simulink library "LnrIntrpnDyn"  (R2013b)
settings: Solver=ode45  StartTime=0.0  StopTime=10.0  RelTol=1e-3
settings Model: Creator=qzwc4r  LastModifiedBy=qzwc4r

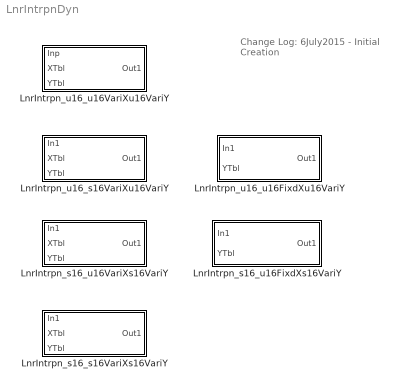
== system LnrIntrpnDyn ==
  note: Change Log:
      |
      | 6July2015
      | - Initial Creation
  LnrIntrpn_s16_s16VariXs16VariY : Subsystem  mask(LnrIntrpn_s16_s16VariXs16VariY){}
      mask help:
      | Linear interpolation with signed input and signed output (variable X axis)
      | XTbl and YTbl sizes must be equal.
      settings: AttributesFormatString=Lnr ( s16VariX , s16VariY )
      mask Display:
      | Xx = [0.3, .9];
      | Xy = [0.5, 0.5];
      | Yx = [0.6, 0.6];
      | Yy = [0.1, .9];
      | 
      | px = [.3, .4, .6, .7, .8, .9];
      | py = [.1,  .1, .25, .4, .5, .9];
      | plot(Xx,Xy, Yx,Yy, px,py)
      | 
      | port_label('input',1,'Inp')
      | port_label('input',2,'XTbl')
      | port_label('input',3,'YTbl')
  LnrIntrpn_s16_u16FixdXs16VariY : Subsystem  mask(LnrIntrpn_s16_u16FixdXs16VariY){DeltaX=[]}
      mask help: Linear interpolation with unsigned input and signed output (fixed X axis)
      settings: AttributesFormatString=Lnr ( u16FixdX , s16VariY )
      mask Display:
      | Xx = [0.3, .9];
      | Xy = [0.4, 0.4];
      | Yx = [0.3, 0.3];
      | Yy = [0, .9];
      | 
      | px = [0.3, .4, .5, .6, .8, .9];
      | py = [.75, .75, .6, .3, .1, .1];
      | 
      | %tic marks
      | tx1 = [0.3, 0.3];
      | tx2 = tx1 + 0.15;
      | tx3 = tx2 + 0.15;
      | tx4 = tx3 + 0.15;
      | tx5 = tx4 + 0.15;
      | ty = [.27, .53];
      | 
      | plot(Xx,Xy, Yx,Yy, px,py, tx1,ty, tx2,ty, tx3,ty, tx4,ty, tx5,ty)
      | 
      | port_label('input',1,'Inp')
      | port_label('input',2,'YTbl')
  LnrIntrpn_s16_u16VariXs16VariY : Subsystem  mask(LnrIntrpn_s16_u16VariXs16VariY){}
      mask help:
      | Linear interpolation with unsigned input and signed output (variable X axis)
      | XTbl and YTbl sizes must be equal.
      settings: AttributesFormatString=Lnr ( u16VariX , s16VariY )
      mask Display:
      | Xx = [0.3, .9];
      | Xy = [0.4, 0.4];
      | Yx = [0.3, 0.3];
      | Yy = [0, .9];
      | 
      | px = [0.3, .35, .4, .6, .8, .9];
      | py = [.75, .75, .7, .3, .1, .1];
      | plot(Xx,Xy, Yx,Yy, px,py)
      | 
      | port_label('input',1,'Inp')
      | port_label('input',2,'XTbl')
      | port_label('input',3,'YTbl')
  LnrIntrpn_u16_s16VariXu16VariY : Subsystem  mask(LnrIntrpn_u16_s16VariXu16VariY){}
      mask help:
      | Linear interpolation with signed input and unsigned output (variable X axis)
      | XTbl and YTbl sizes must be equal.
      settings: AttributesFormatString=Lnr ( s16VariX , u16VariY )
      mask Display:
      | Xx = [0.3, .9];
      | Xy = [.05, .05];
      | Yx = [.6, .6];
      | Yy = [.05, .9];
      | 
      | px = [0.3, .4, .5, .6, .7, .9];
      | py = [.15, .15, .25, .5, .6, .65];
      | plot(Xx,Xy, Yx,Yy, px,py)
      | 
      | port_label('input',1,'Inp')
      | port_label('input',2,'XTbl')
      | port_label('input',3,'YTbl')
  LnrIntrpn_u16_u16FixdXu16VariY : Subsystem  mask(LnrIntrpn_u16_u16FixdXu16VariY){DeltaX=[]}
      mask help: Linear interpolation with unsigned input and unsigned output (fixed X axis)
      settings: AttributesFormatString=Lnr ( u16FixdX , u16VariY )
      mask Display:
      | Xx = [0.3, .9];
      | Xy = [0.1, 0.1];
      | Yx = [0.3, 0.3];
      | Yy = [0.1, .9];
      | 
      | px = [0.3, .35, .4, .45, .5, .6, .8];
      | py = [0.1,  0.4, .6, .7, .75, .78, .8];
      | 
      | %tic marks
      | tx1 = [0.3, 0.3];
      | tx2 = tx1 + 0.15;
      | tx3 = tx2 + 0.15;
      | tx4 = tx3 + 0.15;
      | tx5 = tx4 + 0.15;
      | ty = [.1, .25];
      | 
      | plot(Xx,Xy, Yx,Yy, px,py, tx1,ty, tx2,ty, tx3,ty, tx4,ty, tx5,ty)
      | 
      | port_label('input',1,'Inp')
      | port_label('input',2,'YTbl')
  LnrIntrpn_u16_u16VariXu16VariY : Subsystem  mask(LnrIntrpn_u16_u16VariXu16VariY){}
      mask help:
      | Linear interpolation with unsigned input and unsigned output (variable X axis)
      | XTbl and YTbl sizes must be equal.
      settings: AttributesFormatString=Lnr ( u16VariX , u16VariY )
      mask Display:
      | Xx = [0.25, .9];
      | Xy = [0.1, 0.1];
      | Yx = [0.25, 0.25];
      | Yy = [0.1, .9];
      | 
      | px = [0.25, .3, .35, .4, .5, .6, .8];
      | py = [0.1,  0.4, .6, .7, .75, .78, .8];
      | plot(Xx,Xy, Yx,Yy, px,py)
      | 
      | port_label('input',1,'Inp')
      | port_label('input',2,'XTbl')
      | port_label('input',3,'YTbl')

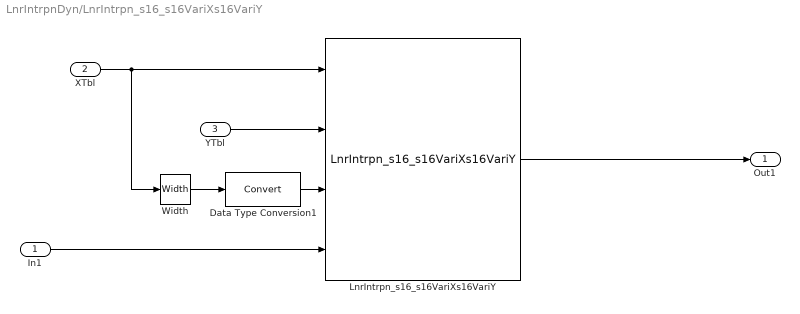
== system LnrIntrpnDyn/LnrIntrpn_s16_s16VariXs16VariY ==
  In1 : Inport
  XTbl : Inport  Port=2
  YTbl : Inport  Port=3
  Data Type Conversion1 : DataTypeConversion
  LnrIntrpn_s16_s16VariXs16VariY : S-Function  FunctionName=LnrIntrpn_s16_s16VariXs16VariY  EnableBusSupport=off  mask(Legacy Function){SFunctionSpec=int16 y1 = LnrIntrpn_s16_s16VariXs16VariY( int16 u1[],  int16 u2[], uint16 u3,  int16 u4), ShowSpec=on}
      mask prompts: ShowSpec "Display function specification"
      mask help:
      | This block allows you to call the legacy functions specified by the following Legacy Code Tool definition:
      | def.SFunctionName = 'LnrIntrpn_s16_s16VariXs16VariY';
      | def.OutputFcnSpec = ' int16 y1 = LnrIntrpn_s16_s16VariXs16VariY( int16 u1[],  int16 u2[], uint16 u3,  int16 u4)';
      | def.HeaderFiles = {'NxtrIntrpn.h', 'NxtrIntrpn_MemMap.h', 'Std_Types.h', 'Platform_Types.h', 'Compiler.h', 'Compiler_Cfg.h'};
      | def.SourceFiles = {'NxtrIntrpn.c'};
      | def.IncPaths = {'..\SrcFiles'};
      | def.SrcPaths = {'..\SrcFiles'};
      mask Help: <p>This block was generated automatically by the Legacy Code Tool. For detailed help on this tool, call<a href="matlab:legacy_code('help')"> legacy_code('help')</a>.</p>
      mask Callback ShowSpec:
      | if strcmp(get_param(gcbh, 'ShowSpec'), 'on')
      |   set_param(gcbh, 'MaskDisplay', sprintf('fprintf(''%s'');', get_param(gcbh, 'SFunctionSpec')));
      | else
      |   set_param(gcbh, 'MaskDisplay', sprintf('fprintf(''%s'');', get_param(gcbh, 'FunctionName')));
      | end
      mask Display: fprintf('%s',' int16 y1 = LnrIntrpn_s16_s16VariXs16VariY( int16 u1[],  int16 u2[], uint16 u3,  int16 u4)');
  Width : Width
  Out1 : Outport
  wires:
  In1/1 -> LnrIntrpn_s16_s16VariXs16VariY/4
  LnrIntrpn_s16_s16VariXs16VariY/1 -> Out1/1
  YTbl/1 -> LnrIntrpn_s16_s16VariXs16VariY/2
  Width/1 -> Data Type Conversion1/1
  XTbl/1 -> Width/1, LnrIntrpn_s16_s16VariXs16VariY/1
  Data Type Conversion1/1 -> LnrIntrpn_s16_s16VariXs16VariY/3

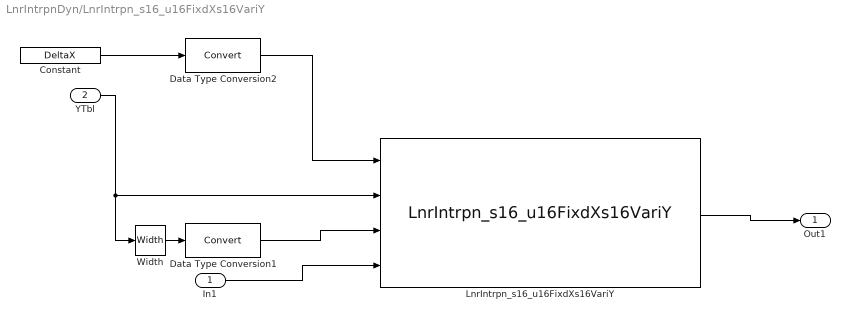
== system LnrIntrpnDyn/LnrIntrpn_s16_u16FixdXs16VariY ==
  In1 : Inport
  YTbl : Inport  Port=2
  Constant : Constant  Value=DeltaX
  Data Type Conversion1 : DataTypeConversion
  Data Type Conversion2 : DataTypeConversion
  LnrIntrpn_s16_u16FixdXs16VariY : S-Function  FunctionName=LnrIntrpn_s16_u16FixdXs16VariY  EnableBusSupport=off  mask(Legacy Function){SFunctionSpec=int16 y1 = LnrIntrpn_s16_u16FixdXs16VariY(uint16 u1,  int16 u2[], uint16 u3, uint16 u4), ShowSpec=on}
      mask prompts: ShowSpec "Display function specification"
      mask help:
      | This block allows you to call the legacy functions specified by the following Legacy Code Tool definition:
      | def.SFunctionName = 'LnrIntrpn_s16_u16FixdXs16VariY';
      | def.OutputFcnSpec = ' int16 y1 = LnrIntrpn_s16_u16FixdXs16VariY(uint16 u1,  int16 u2[], uint16 u3, uint16 u4)';
      | def.HeaderFiles = {'NxtrIntrpn.h', 'NxtrIntrpn_MemMap.h', 'Std_Types.h', 'Platform_Types.h', 'Compiler.h', 'Compiler_Cfg.h'};
      | def.SourceFiles = {'NxtrIntrpn.c'};
      | def.IncPaths = {'..\SrcFiles'};
      | def.SrcPaths = {'..\SrcFiles'};
      mask Help: <p>This block was generated automatically by the Legacy Code Tool. For detailed help on this tool, call<a href="matlab:legacy_code('help')"> legacy_code('help')</a>.</p>
      mask Callback ShowSpec:
      | if strcmp(get_param(gcbh, 'ShowSpec'), 'on')
      |   set_param(gcbh, 'MaskDisplay', sprintf('fprintf(''%s'');', get_param(gcbh, 'SFunctionSpec')));
      | else
      |   set_param(gcbh, 'MaskDisplay', sprintf('fprintf(''%s'');', get_param(gcbh, 'FunctionName')));
      | end
      mask Display: fprintf('%s',' int16 y1 = LnrIntrpn_s16_u16FixdXs16VariY(uint16 u1,  int16 u2[], uint16 u3, uint16 u4)');
  Width : Width
  Out1 : Outport
  wires:
  LnrIntrpn_s16_u16FixdXs16VariY/1 -> Out1/1
  YTbl/1 -> Width/1, LnrIntrpn_s16_u16FixdXs16VariY/2
  Constant/1 -> Data Type Conversion2/1
  Width/1 -> Data Type Conversion1/1
  In1/1 -> LnrIntrpn_s16_u16FixdXs16VariY/4
  Data Type Conversion1/1 -> LnrIntrpn_s16_u16FixdXs16VariY/3
  Data Type Conversion2/1 -> LnrIntrpn_s16_u16FixdXs16VariY/1

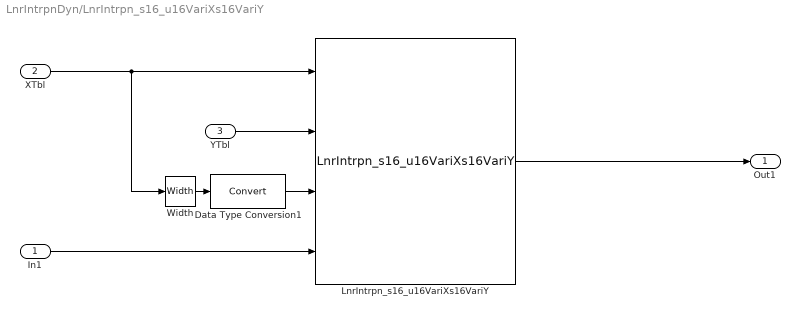
== system LnrIntrpnDyn/LnrIntrpn_s16_u16VariXs16VariY ==
  In1 : Inport
  XTbl : Inport  Port=2
  YTbl : Inport  Port=3
  Data Type Conversion1 : DataTypeConversion
  LnrIntrpn_s16_u16VariXs16VariY : S-Function  FunctionName=LnrIntrpn_s16_u16VariXs16VariY  EnableBusSupport=off  mask(Legacy Function){SFunctionSpec=int16 y1 = LnrIntrpn_s16_u16VariXs16VariY(uint16 u1[],  int16 u2[], uint16 u3, uint16 u4), ShowSpec=on}
      mask prompts: ShowSpec "Display function specification"
      mask help:
      | This block allows you to call the legacy functions specified by the following Legacy Code Tool definition:
      | def.SFunctionName = 'LnrIntrpn_s16_u16VariXs16VariY';
      | def.OutputFcnSpec = ' int16 y1 = LnrIntrpn_s16_u16VariXs16VariY(uint16 u1[],  int16 u2[], uint16 u3, uint16 u4)';
      | def.HeaderFiles = {'NxtrIntrpn.h', 'NxtrIntrpn_MemMap.h', 'Std_Types.h', 'Platform_Types.h', 'Compiler.h', 'Compiler_Cfg.h'};
      | def.SourceFiles = {'NxtrIntrpn.c'};
      | def.IncPaths = {'..\SrcFiles'};
      | def.SrcPaths = {'..\SrcFiles'};
      mask Help: <p>This block was generated automatically by the Legacy Code Tool. For detailed help on this tool, call<a href="matlab:legacy_code('help')"> legacy_code('help')</a>.</p>
      mask Callback ShowSpec:
      | if strcmp(get_param(gcbh, 'ShowSpec'), 'on')
      |   set_param(gcbh, 'MaskDisplay', sprintf('fprintf(''%s'');', get_param(gcbh, 'SFunctionSpec')));
      | else
      |   set_param(gcbh, 'MaskDisplay', sprintf('fprintf(''%s'');', get_param(gcbh, 'FunctionName')));
      | end
      mask Display: fprintf('%s',' int16 y1 = LnrIntrpn_s16_u16VariXs16VariY(uint16 u1[],  int16 u2[], uint16 u3, uint16 u4)');
  Width : Width
  Out1 : Outport
  wires:
  XTbl/1 -> Width/1, LnrIntrpn_s16_u16VariXs16VariY/1
  Width/1 -> Data Type Conversion1/1
  YTbl/1 -> LnrIntrpn_s16_u16VariXs16VariY/2
  LnrIntrpn_s16_u16VariXs16VariY/1 -> Out1/1
  In1/1 -> LnrIntrpn_s16_u16VariXs16VariY/4
  Data Type Conversion1/1 -> LnrIntrpn_s16_u16VariXs16VariY/3

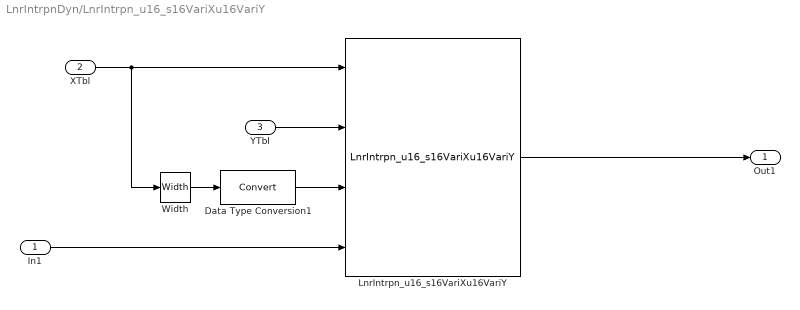
== system LnrIntrpnDyn/LnrIntrpn_u16_s16VariXu16VariY ==
  In1 : Inport
  XTbl : Inport  Port=2
  YTbl : Inport  Port=3
  Data Type Conversion1 : DataTypeConversion
  LnrIntrpn_u16_s16VariXu16VariY : S-Function  FunctionName=LnrIntrpn_u16_s16VariXu16VariY  EnableBusSupport=off  mask(Legacy Function){SFunctionSpec=uint16 y1 = LnrIntrpn_u16_s16VariXu16VariY( int16 u1[], uint16 u2[], uint16 u3,  int16 u4), ShowSpec=on}
      mask prompts: ShowSpec "Display function specification"
      mask help:
      | This block allows you to call the legacy functions specified by the following Legacy Code Tool definition:
      | def.SFunctionName = 'LnrIntrpn_u16_s16VariXu16VariY';
      | def.OutputFcnSpec = 'uint16 y1 = LnrIntrpn_u16_s16VariXu16VariY( int16 u1[], uint16 u2[], uint16 u3,  int16 u4)';
      | def.HeaderFiles = {'NxtrIntrpn.h', 'NxtrIntrpn_MemMap.h', 'Std_Types.h', 'Platform_Types.h', 'Compiler.h', 'Compiler_Cfg.h'};
      | def.SourceFiles = {'NxtrIntrpn.c'};
      | def.IncPaths = {'..\SrcFiles'};
      | def.SrcPaths = {'..\SrcFiles'};
      mask Help: <p>This block was generated automatically by the Legacy Code Tool. For detailed help on this tool, call<a href="matlab:legacy_code('help')"> legacy_code('help')</a>.</p>
      mask Callback ShowSpec:
      | if strcmp(get_param(gcbh, 'ShowSpec'), 'on')
      |   set_param(gcbh, 'MaskDisplay', sprintf('fprintf(''%s'');', get_param(gcbh, 'SFunctionSpec')));
      | else
      |   set_param(gcbh, 'MaskDisplay', sprintf('fprintf(''%s'');', get_param(gcbh, 'FunctionName')));
      | end
      mask Display: fprintf('%s','uint16 y1 = LnrIntrpn_u16_s16VariXu16VariY( int16 u1[], uint16 u2[], uint16 u3,  int16 u4)');
  Width : Width
  Out1 : Outport
  wires:
  XTbl/1 -> Width/1, LnrIntrpn_u16_s16VariXu16VariY/1
  Width/1 -> Data Type Conversion1/1
  YTbl/1 -> LnrIntrpn_u16_s16VariXu16VariY/2
  LnrIntrpn_u16_s16VariXu16VariY/1 -> Out1/1
  In1/1 -> LnrIntrpn_u16_s16VariXu16VariY/4
  Data Type Conversion1/1 -> LnrIntrpn_u16_s16VariXu16VariY/3

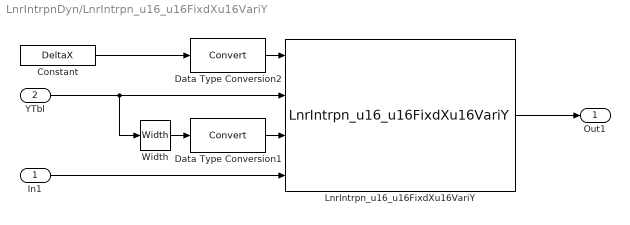
== system LnrIntrpnDyn/LnrIntrpn_u16_u16FixdXu16VariY ==
  In1 : Inport
  YTbl : Inport  Port=2
  Constant : Constant  Value=DeltaX
  Data Type Conversion1 : DataTypeConversion
  Data Type Conversion2 : DataTypeConversion
  LnrIntrpn_u16_u16FixdXu16VariY : S-Function  FunctionName=LnrIntrpn_u16_u16FixdXu16VariY  EnableBusSupport=off  mask(Legacy Function){SFunctionSpec=uint16 y1 = LnrIntrpn_u16_u16FixdXu16VariY(uint16 u1, uint16 u2[], uint16 u3, uint16 u4), ShowSpec=on}
      mask prompts: ShowSpec "Display function specification"
      mask help:
      | This block allows you to call the legacy functions specified by the following Legacy Code Tool definition:
      | def.SFunctionName = 'LnrIntrpn_u16_u16FixdXu16VariY';
      | def.OutputFcnSpec = 'uint16 y1 = LnrIntrpn_u16_u16FixdXu16VariY(uint16 u1, uint16 u2[], uint16 u3, uint16 u4)';
      | def.HeaderFiles = {'NxtrIntrpn.h', 'NxtrIntrpn_MemMap.h', 'Std_Types.h', 'Platform_Types.h', 'Compiler.h', 'Compiler_Cfg.h'};
      | def.SourceFiles = {'NxtrIntrpn.c'};
      | def.IncPaths = {'..\SrcFiles'};
      | def.SrcPaths = {'..\SrcFiles'};
      mask Help: <p>This block was generated automatically by the Legacy Code Tool. For detailed help on this tool, call<a href="matlab:legacy_code('help')"> legacy_code('help')</a>.</p>
      mask Callback ShowSpec:
      | if strcmp(get_param(gcbh, 'ShowSpec'), 'on')
      |   set_param(gcbh, 'MaskDisplay', sprintf('fprintf(''%s'');', get_param(gcbh, 'SFunctionSpec')));
      | else
      |   set_param(gcbh, 'MaskDisplay', sprintf('fprintf(''%s'');', get_param(gcbh, 'FunctionName')));
      | end
      mask Display: fprintf('uint16 y1 = LnrIntrpn_u16_u16FixdXu16VariY(uint16 u1, uint16 u2[], uint16 u3, uint16 u4)');
  Width : Width
  Out1 : Outport
  wires:
  Width/1 -> Data Type Conversion1/1
  YTbl/1 -> Width/1, LnrIntrpn_u16_u16FixdXu16VariY/2
  Constant/1 -> Data Type Conversion2/1
  In1/1 -> LnrIntrpn_u16_u16FixdXu16VariY/4
  LnrIntrpn_u16_u16FixdXu16VariY/1 -> Out1/1
  Data Type Conversion1/1 -> LnrIntrpn_u16_u16FixdXu16VariY/3
  Data Type Conversion2/1 -> LnrIntrpn_u16_u16FixdXu16VariY/1

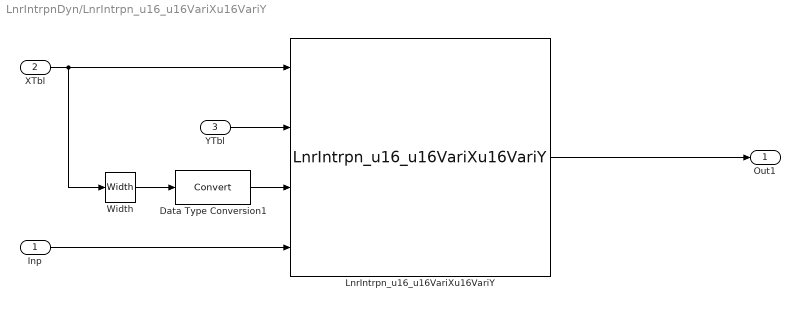
== system LnrIntrpnDyn/LnrIntrpn_u16_u16VariXu16VariY ==
  Inp : Inport
  XTbl : Inport  Port=2
  YTbl : Inport  Port=3
  Data Type Conversion1 : DataTypeConversion
  LnrIntrpn_u16_u16VariXu16VariY : S-Function  FunctionName=LnrIntrpn_u16_u16VariXu16VariY  EnableBusSupport=off  mask(Legacy Function){SFunctionSpec=uint16 y1 = LnrIntrpn_u16_u16VariXu16VariY(uint16 u1[], uint16 u2[], uint16 u3, uint16 u4), ShowSpec=on}
      mask prompts: ShowSpec "Display function specification"
      mask help:
      | This block allows you to call the legacy functions specified by the following Legacy Code Tool definition:
      | def.SFunctionName = 'LnrIntrpn_u16_u16VariXu16VariY';
      | def.OutputFcnSpec = 'uint16 y1 = LnrIntrpn_u16_u16VariXu16VariY(uint16 u1[], uint16 u2[], uint16 u3, uint16 u4)';
      | def.HeaderFiles = {'NxtrIntrpn.h', 'NxtrIntrpn_MemMap.h', 'Std_Types.h', 'Platform_Types.h', 'Compiler.h', 'Compiler_Cfg.h'};
      | def.SourceFiles = {'NxtrIntrpn.c'};
      | def.IncPaths = {'..\SrcFiles'};
      | def.SrcPaths = {'..\SrcFiles'};
      mask Help: <p>This block was generated automatically by the Legacy Code Tool. For detailed help on this tool, call<a href="matlab:legacy_code('help')"> legacy_code('help')</a>.</p>
      mask Callback ShowSpec:
      | if strcmp(get_param(gcbh, 'ShowSpec'), 'on')
      |   set_param(gcbh, 'MaskDisplay', sprintf('fprintf(''%s'');', get_param(gcbh, 'SFunctionSpec')));
      | else
      |   set_param(gcbh, 'MaskDisplay', sprintf('fprintf(''%s'');', get_param(gcbh, 'FunctionName')));
      | end
      mask Display: fprintf('%s','uint16 y1 = LnrIntrpn_u16_u16VariXu16VariY(uint16 u1[], uint16 u2[], uint16 u3, uint16 u4)');
  Width : Width
  Out1 : Outport
  wires:
  Inp/1 -> LnrIntrpn_u16_u16VariXu16VariY/4
  LnrIntrpn_u16_u16VariXu16VariY/1 -> Out1/1
  YTbl/1 -> LnrIntrpn_u16_u16VariXu16VariY/2
  Width/1 -> Data Type Conversion1/1
  XTbl/1 -> LnrIntrpn_u16_u16VariXu16VariY/1, Width/1
  Data Type Conversion1/1 -> LnrIntrpn_u16_u16VariXu16VariY/3
